simulink model "P2_linealizado"  (R2017a)
settings: Solver=VariableStepAuto  StartTime=0.0  StopTime=10.0  RelTol=1e-3
values from neighbouring files (symbols this model uses):
  b = 0.5    [P2_comparacion.m]    (also in P2_script_lineal.m; P2_script_no_lineal.m; mrm.m = 8)
  i_eq = 0.5    [P2_comparacion.m]    (also in P2_script_lineal.m)
  Ki = (2*K*i_eq)/(y_eq)    (= 7.8400627205)    [P2_comparacion.m]    (also in P2_script_lineal.m)
  Ky = -(K*(i_eq)^2)/((y_eq)^2)    (= -7.68332293268)    [P2_comparacion.m]    (also in P2_script_lineal.m)
  L = 0.01    [P2_comparacion.m]    (also in P2_script_lineal.m; P2_script_no_lineal.m)
  M = 0.2    [P2_comparacion.m]    (also in P2_script_lineal.m; P2_script_no_lineal.m)
  R = 20    [P2_comparacion.m]    (also in P2_script_lineal.m; P2_script_no_lineal.m)
  u_eq = 10    [P2_comparacion.m]    (also in P2_script_lineal.m)
  y_eq = 0.2551    [P2_comparacion.m]    (also in P2_script_lineal.m)
settings Model: Creator=joaqu  LastModifiedBy=joaqu

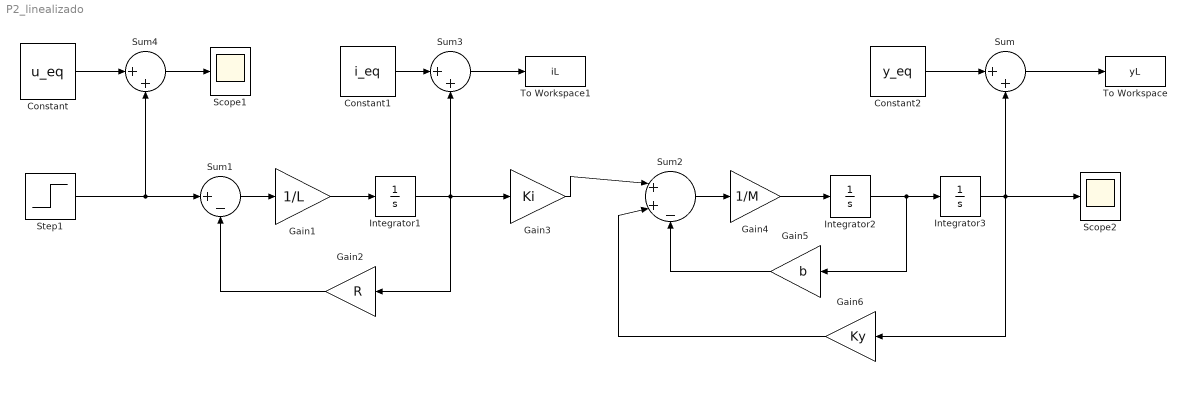
== system P2_linealizado ==
  Constant : Constant  Value=u_eq
  Constant1 : Constant  Value=i_eq
  Constant2 : Constant  Value=y_eq
  Gain1 : Gain  Gain=1/L
  Gain2 : Gain  Gain=R
  Gain3 : Gain  Gain=Ki
  Gain4 : Gain  Gain=1/M
  Gain5 : Gain  Gain=b
  Gain6 : Gain  Gain=Ky
  Integrator1 : Integrator
  Integrator2 : Integrator
  Integrator3 : Integrator
  Scope1 : Scope
  Scope2 : Scope
  Step1 : Step  Time=0  After=0.2  SampleTime=0
  Sum : Sum  Inputs=|++
  Sum1 : Sum  Inputs=|+-
  Sum2 : Sum  Inputs=|++-
  Sum3 : Sum  Inputs=|++
  Sum4 : Sum  Inputs=|++
  To Workspace : ToWorkspace  VariableName=yL  SaveFormat=Timeseries  SampleTime=-1
  To Workspace1 : ToWorkspace  VariableName=iL  SaveFormat=Timeseries  SampleTime=-1
  wires:
  Step1/1 -> Sum1/1, Sum4/2
  Sum1/1 -> Gain1/1
  Gain1/1 -> Integrator1/1
  Integrator1/1 -> Gain3/1, Sum3/2, Gain2/1
  Gain2/1 -> Sum1/2
  Gain3/1 -> Sum2/1
  Sum2/1 -> Gain4/1
  Gain4/1 -> Integrator2/1
  Integrator2/1 -> Integrator3/1, Gain5/1
  Integrator3/1 -> Scope2/1, Sum/2, Gain6/1
  Gain6/1 -> Sum2/2
  Constant/1 -> Sum4/1
  Sum4/1 -> Scope1/1
  Constant1/1 -> Sum3/1
  Sum3/1 -> To Workspace1/1
  Constant2/1 -> Sum/1
  Gain5/1 -> Sum2/3
  Sum/1 -> To Workspace/1
